simulink model "chap10_4sim"  (Simulink 3.00)
settings: Solver=ode45  StartTime=0.0  StopTime=10  FixedStep=0.00000010  RelTol=1e-3
settings Model: LastModifiedBy=liu

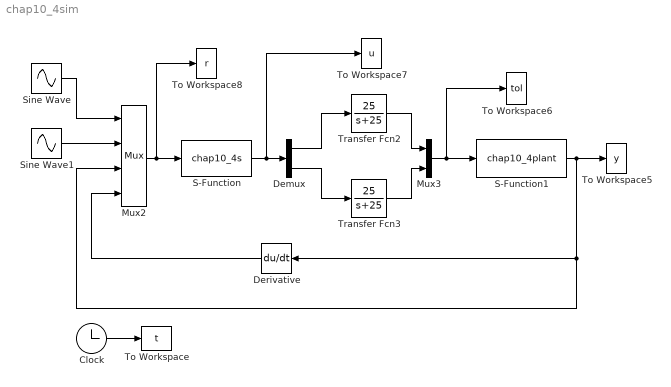
== system chap10_4sim ==
  Clock : Clock
  Demux : Demux  Outputs=2
  Derivative : Derivative  Orientation=left
  Mux2 : Mux  Inputs=4
      settings: DisplayOption=none
  Mux3 : Mux  Inputs=2
  S-Function : S-Function  FunctionName=chap10_4s  PortCounts=[]  SFunctionModules=''
  S-Function1 : S-Function  FunctionName=chap10_4plant  PortCounts=[]  SFunctionModules=''
  Sine Wave : Sin  Amplitude=1  Frequency=pi  Phase=0  SampleTime=0
  Sine Wave1 : Sin  Amplitude=1  Frequency=pi  Phase=pi/2  SampleTime=0
  To Workspace : ToWorkspace  VariableName=t  SampleTime=-1  SaveFormat=Matrix
  To Workspace5 : ToWorkspace  VariableName=y  SampleTime=-1  SaveFormat=Matrix
  To Workspace6 : ToWorkspace  VariableName=tol  SampleTime=-1  SaveFormat=Matrix
  To Workspace7 : ToWorkspace  VariableName=u  SampleTime=-1  SaveFormat=Matrix
  To Workspace8 : ToWorkspace  VariableName=r  SampleTime=-1  SaveFormat=Matrix
  Transfer Fcn2 : TransferFcn  Numerator=[25]  Denominator=[1 25]
  Transfer Fcn3 : TransferFcn  Numerator=[25]  Denominator=[1 25]
  wires:
  Demux/2 -> Transfer Fcn3/1
  Transfer Fcn3/1 -> Mux3/2
  Transfer Fcn2/1 -> Mux3/1
  Demux/1 -> Transfer Fcn2/1
  S-Function1/1 -> To Workspace5/1, Derivative/1, Mux2/3
  S-Function/1 -> Demux/1, To Workspace7/1
  Mux3/1 -> S-Function1/1, To Workspace6/1
  Derivative/1 -> Mux2/4
  Sine Wave/1 -> Mux2/1
  Sine Wave1/1 -> Mux2/2
  Clock/1 -> To Workspace/1
  Mux2/1 -> S-Function/1, To Workspace8/1
